simulink model "VU_lineFollow1"  (Simulink 7.5)
settings: Solver=FixedStepDiscrete  StartTime=0.0  StopTime=inf  FixedStep=0.1  RelTol=1e-3
libraries: lego_nxt_lib x4
settings Model: Creator=jpeytonj  LastModifiedBy=jpeytonj
settings RTWCC: SystemTargetFile=lrt.tlc  GenCodeOnly=on  TemplateMakefile=lrt_ecrobot.tmf  Description=Lego NXT Real-Time Target  ProcessScript=lrt_make_rtw_hook
settings STFCustomTargetCC: ModelReferenceCompliant=off  GeneratePreprocessorConditionals=Disable all  MatFileLogging=on  SystemTargetFile=lrt.tlc
settings GRTTargetCC: ModelReferenceCompliant=off  ParMdlRefBuildCompliant=off  CompOptLevelCompliant=off  ExtModeMexFile=noextcomm
settings CustomProperty: DataType=RTWOptions_EnumType_C__RTtools_VU-LRT_lrt_1codeGenType  Value=Integer-only
settings EnumStrPairs: String=Integer-only

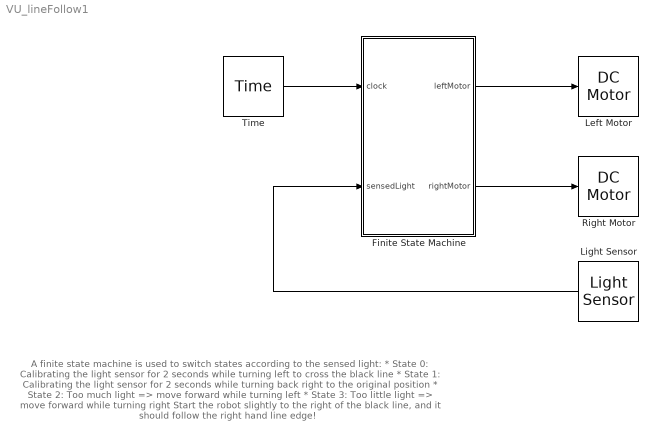
== system VU_lineFollow1 ==
  note: A finite state machine is used to switch states according to the sensed light:
      | * State 0:  Calibrating the light sensor for 2 seconds while turning left to cross the black line
      | * State 1:  Calibrating the light sensor for 2 seconds while turning back right to the original position
      | * State 2:  Too much light => move forward while turning left
      | * State 3:  Too little light => move forward while turning right
      | Start the robot slightly to the right of the black line, and it should follow the right hand line edge!
  Finite State Machine : Stateflow chart  TreatAsAtomicUnit=on
  Left Motor : lego_nxt_lib/DC Motor  port=Port C  brake=Coast
  Light Sensor : lego_nxt_lib/Light Sensor  port=Port 3  st=0.1
  Right Motor : lego_nxt_lib/DC Motor  port=Port B  brake=Coast
  Time : lego_nxt_lib/Time  st=0.1
  wires:
  Finite State Machine/1(leftMotor) -> Left Motor/1
  Finite State Machine/2(rightMotor) -> Right Motor/1
  Light Sensor/1 -> Finite State Machine/2(sensedLight)
  Time/1 -> Finite State Machine/1(clock)

== matlab function Finite State Machine ==
  data: clock input double; sensedLight input double; leftMotor output double; rightMotor output double
function [leftMotor, rightMotor] = fsm(clock, sensedLight)

persistent currentState maxLight minLight threshold 

if isempty(currentState),
    currentState= uint8(0);
    maxLight= uint16(0);
    minLight= uint16(1023);
    threshold= uint16(45);
end;

leftMotor= int8(0);
rightMotor= int8(0);

switch currentState
    case 0 %Calibration - turning left
        leftMotor= int8(-60);
        rightMotor= int8(60);
        if sensedLight>maxLight, maxLight= sensedLight; end;
        if sensedLight<minLight, minLight= sensedLight; end;
        if (clock>2000), currentState= uint8(1); end;
    case 1 %Calibration - turning right
        leftMotor= int8(60);
        rightMotor= int8(-60);
        if sensedLight>maxLight, maxLight= sensedLight; end;
        if sensedLight<minLight, minLight= sensedLight; end;
        if (clock>4000), 
            threshold = (maxLight + minLight)/2;
            currentState= uint8(2); 
        end;
    case 2 %Too much light => turn Left
        leftMotor= int8(55);
        rightMotor= int8(65);
        if sensedLight<threshold, currentState= uint8(3); end;
    case 3 %Too little light => turn Right
        leftMotor= int8(65);
        rightMotor= int8(55);
        if sensedLight>threshold, currentState= uint8(2); end;
end
